simulink model "pid_controller_pitch"  (R2023a)
settings: Solver=FixedStepAuto  StartTime=0.0  StopTime=inf  FixedStep=Ts_slk  RelTol=1e-3  EnableMultiTasking=on
undefined symbols (not defined in the file): A_cond, B_cond, C, D, dev, IMU_w_b_bias, K, Main, meas_pole, P0_phth, P0_ps, prefilter_pole, pwm_output0, Q_phth, q_ps, R_phth, r_ps, Rz, Ts_EKF_integr, Ts_EKF_meas, Ts_slk, x0_phth, x0_ps
libraries: px4Sensorslib x4, slpidlib x2, cstblocks x1, px4lib x1, px4uORBlib x1, sharedtransform x1
(part 1 of 2)
settings Model: ExtModeTrigDuration=10  Creator=ArriGE66  LastModifiedBy=User
settings SolverCC: PositivePriorityOrder=on
settings OptimizationCC: EnhancedBackFolding=on  PassReuseOutputArgsAs=Individual arguments  ZeroExternalMemoryAtStartup=off  ZeroInternalMemoryAtStartup=off  MaxStackSize=64  OptimizeBlockOrder=speed  DifferentSizesBufferReuse=on  OptimizationCustomize=off  EfficientTunableParamExpr=on
settings DebuggingCC: ParameterTunabilityLossMsg=error
settings HardwareCC: ProdBitPerPointer=32  ProdBitPerSizeT=32  ProdBitPerPtrDiffT=32  ProdLargestAtomicInteger=Long  ProdLargestAtomicFloat=Double  ProdWordSize=32  ProdLongLongMode=on  ProdHWDeviceType=ARM Compatible->ARM Cortex
settings SFSimCC: MATLABDynamicMemAlloc=off  SimTargetLang=C++
settings RTWCC: Description=Embedded Coder  SystemTargetFile=ert.tlc  HardwareBoard=PX4 Cube Orange  TLCOptions="-aInlineSetEventsForThisBaseRateFcn=TLC_FALSE -aSuppressMultiTaskScheduler=TLC_FALSE  -aRateBasedStepFcn=0"  TemplateMakefile=ert_default_tmf  Toolchain=GNU Tools for PX4 Autopilots  TargetLang=C++
settings CodeAppCC: ForceParamTrailComments=on  IgnoreCustomStorageClasses=off  OperatorAnnotations=on  SimulinkDataObjDesc=on  SFDataObjDesc=on  InsertBlockDesc=on
settings ERTTargetCC: ExtModeTransport=3  ExtModeStaticAlloc=on  ExtModeStaticAllocSize=1024  ExtModeMexFile=ext_xcp  ExtModeIntrfLevel=Level2 - Open

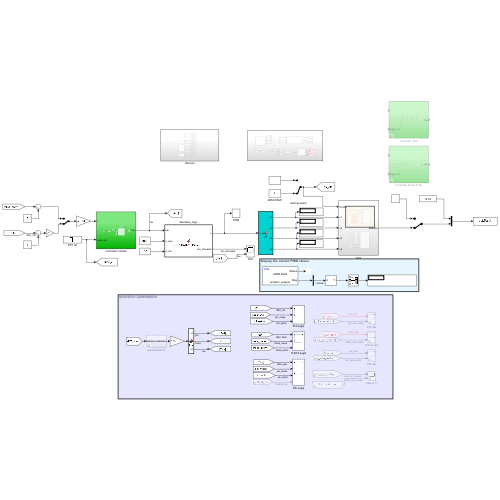
[thumbnail: Simulink's stored preview of the top-level diagram]
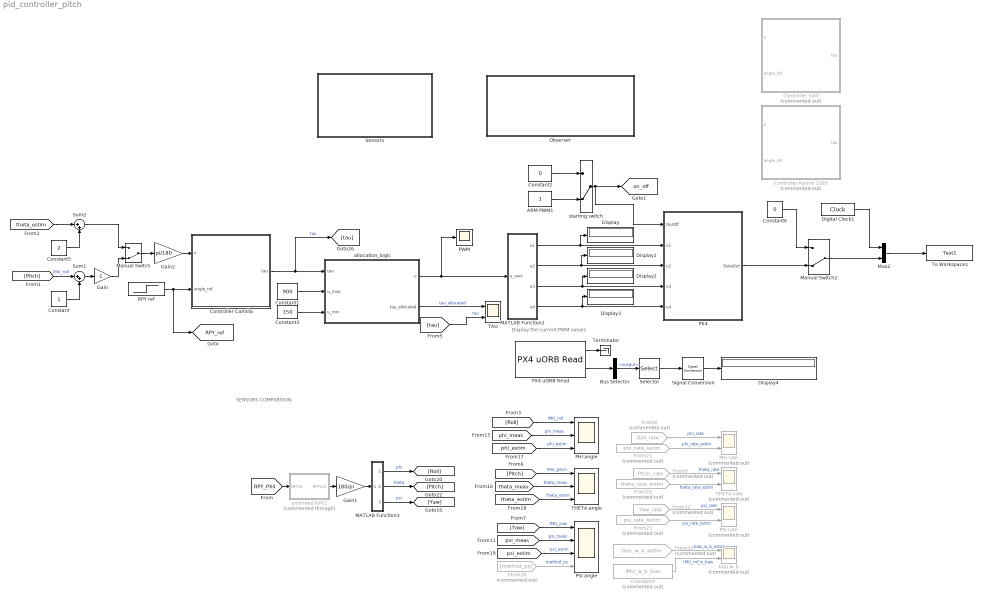
== system pid_controller_pitch ==
  note: Display the current PWM values
  note: SENSORS COMPARISON
  ARM PWM1 : Constant  OutDataTypeStr=boolean  SampleTime=Ts_slk
  Bus Selector : BusSelector  OutputSignals=output
  Constant : Constant  SampleTime=0.01
  Constant1 : Constant  Value=900  SampleTime=0.01
  Constant2 : Constant  Value=0  OutDataTypeStr=boolean
  Constant3 : Constant  Value=150  SampleTime=0.01
  Constant4 : Constant  Commented=on  Value=IMU_w_b_bias
  Constant5 : Constant  Value=2  SampleTime=0.01
  Constant6 : Constant  Value=0  OutDataTypeStr=boolean
  Controller 1dof : Subsystem  Commented=on
  Controller Camilla : Subsystem
  Controller Karimi 2105 : Subsystem  Commented=on
  Digital Clock1 : DigitalClock  SampleTime=0.01
  Display{,1..4} (5 alike) : Display
  From12 : From  Commented=on  GotoTag=Yaw_rate  TagVisibility=global
  From20 : From  Commented=on  GotoTag=method_ps
  From21 : From  Commented=on  GotoTag=phi_rate_estim
  From22 : From  Commented=on  GotoTag=theta_rate_estim
  From23 : From  Commented=on  GotoTag=psi_rate_estim
  From24 : From  Commented=on  GotoTag=bias_w_b_estim
  From8 : From  Commented=on  GotoTag=Roll_rate  TagVisibility=global
  From9 : From  Commented=on  GotoTag=Pitch_rate  TagVisibility=global
  Gain : Gain  Gain=-1
  Gain1 : Gain  Gain=180/pi
  Gain2 : Gain  Gain=pi/180
  MATLAB Function2 : MATLAB Function  TreatAsAtomicUnit=on
  MATLAB Function3 : MATLAB Function  TreatAsAtomicUnit=on
  Manual Switch : ManualSwitch  CurrentSetting=0
  Manual Switch2 : ManualSwitch  CurrentSetting=0
  Mux2 : Mux  Inputs=2
  Observer : Subsystem
  PHI angle : Scope  NumInputPorts=3
  PHI rate : Scope  Commented=on  NumInputPorts=2
  PSI angle : Scope  NumInputPorts=4
  PSI rate : Scope  Commented=on  NumInputPorts=2
  PWM : Scope
  PX4 : Subsystem
  PX4 uORB Read : px4uORBlib/PX4 uORB Read  uORBTopic=actuator_outputs  selectInstance=actuator_outputs  SampleTime=0.01  BlockingMode=off  BlockTimeout=1e-3
  RPY ref : Step  Time=0  After=pi/180*(-4)  SampleTime=Ts_slk
  Selector : Selector  InputPortWidth=16  IndexOptions=Index vector (dialog)  Indices=[1 2 3 4]  OutputSizes=1
  Sensors : Subsystem
  Signal Conversion : SignalConversion  OverrideOpt=off
  Sum1 : Sum  Inputs=|++
  Sum2 : Sum  Inputs=|++
  TAU : Scope  NumInputPorts=2
  THETA angle : Scope  NumInputPorts=3
  THETA rate : Scope  Commented=on  NumInputPorts=2
  Terminator : Terminator
  To Workspace1 : ToWorkspace  VariableName=Test1  SampleTime=-1
      settings: Save2DSignal=2-D array (concatenate along first dimension)
  allocation_logic : MATLAB Function  TreatAsAtomicUnit=on
  bias w_b : Scope  Commented=on  NumInputPorts=2
  starting switch : ManualSwitch  CurrentSetting=0
  unlimited RPY2 : Subsystem  Commented=through
  tag scope: RPY_ref=global, on_off=global
  wires:
  Manual Switch/1 -> Gain2/1
  MATLAB Function2/4(u4) -> PX4/5(u4), Display3/1
  Constant5/1 -> Sum2/2
  Constant4/1 -> bias w_b/2  "IMU_mf_b_bias"
  From8/1 -> PHI rate/1  "phi_rate"
  [RPY_PX4] -> unlimited RPY2/1(RPYin)
  Constant1/1 -> allocation_logic/2(u_max)
  PX4/1(DataOut) -> Manual Switch2/2
  Constant/1 -> Sum1/2
  PX4 uORB Read/2 -> Bus Selector/1
  From22/1 -> THETA rate/2  "theta_rate_estim"
  RPY ref/1 -> [RPY_ref], Controller Camilla/2(angle_ref)
  [theta_estim] -> Sum2/1
  allocation_logic/1(u) -> PWM/1, MATLAB Function2/1(u_vect)
  From21/1 -> PHI rate/2  "phi_rate_estim"
  [phi_meas] -> PHI angle/2  "phi_meas"
  [theta_meas] -> THETA angle/2  "theta_meas"
  unlimited RPY2/1(RPYout) -> Gain1/1
  Constant6/1 -> Manual Switch2/1
  [Roll] -> PHI angle/1  "IMU_roll"
  From23/1 -> PSI rate/2  "psi_rate_estim"
  Selector/1 -> Signal Conversion/1
  [psi_estim] -> PSI angle/3  "psi_estim"
  [theta_estim] -> THETA angle/3  "theta_estim"
  MATLAB Function3/2(y2) -> [Pitch]  "theta"
  Manual Switch2/1 -> Mux2/2
  Sum2/1 -> Manual Switch/1
  [psi_meas] -> PSI angle/2  "psi_meas"
  From20/1 -> PSI angle/4  "method_ps"
  [phi_estim] -> PHI angle/3  "phi_estim"
  Signal Conversion/1 -> Display4/1
  Bus Selector/1 -> Selector/1  "<output>"
  starting switch/1 -> PX4/1(On/Off), [on_off]
  [Pitch] -> THETA angle/1  "IMU_pitch"
  [Yaw] -> PSI angle/1  "IMU_yaw"
  MATLAB Function2/3(u3) -> PX4/4(u3), Display2/1
  From9/1 -> THETA rate/1  "theta_rate"
  Controller Camilla/1(tau) -> [tau], allocation_logic/1(tau)  "tau"
  ARM PWM1/1 -> starting switch/2
  Mux2/1 -> To Workspace1/1
  MATLAB Function3/3(y3) -> [Yaw]  "psi"
  Gain1/1 -> MATLAB Function3/1(u)
  MATLAB Function2/1(u1) -> Display/1, PX4/2(u1)
  [Pitch] -> Sum1/1  "IMU_roll"
  From12/1 -> PSI rate/1  "psi_rate"
  Digital Clock1/1 -> Mux2/1
  allocation_logic/2(tau_allocated) -> TAU/1  "tau_allocated"
  MATLAB Function3/1(y1) -> [Roll]  "phi"
  Sum1/1 -> Gain/1
  Constant3/1 -> allocation_logic/3(u_min)
  [tau] -> TAU/2  "tau"
  MATLAB Function2/2(u2) -> Display1/1, PX4/3(u2)
  From24/1 -> bias w_b/1  "bias_w_b_estim"
  Gain2/1 -> Controller Camilla/1(x)
  Constant2/1 -> starting switch/1
  PX4 uORB Read/1 -> Terminator/1
  Gain/1 -> Manual Switch/2

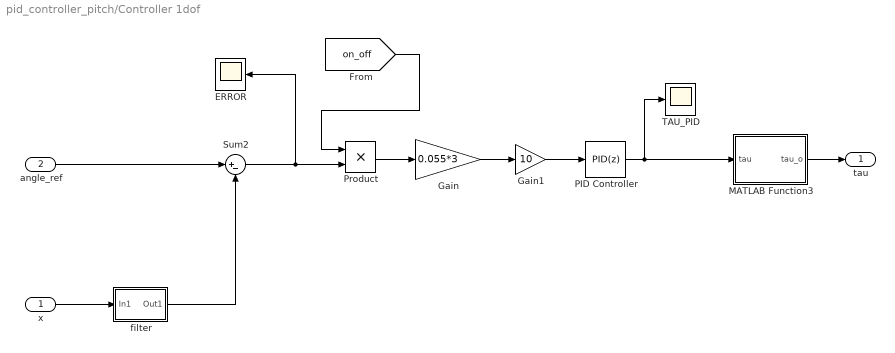
== system pid_controller_pitch/Controller 1dof ==
  x : Inport
  angle_ref : Inport  Port=2
  ERROR : Scope
  Gain : Gain  Gain=0.055*3
  Gain1 : Gain  Gain=10
  MATLAB Function3 : MATLAB Function  TreatAsAtomicUnit=on
  PID Controller : slpidlib/PID Controller  Controller=PID  Form=Parallel  TimeDomain=Discrete-time  UseExternalTs=off  SampleTime=Ts_slk  IntegratorMethod=Forward Euler  FilterMethod=Forward Euler  ControllerParametersSource=internal  P=0.01  I=0  UseKiTs=off  D=1  N=100  UseFilter=on  TunerSelectOption=Transfer Function Based (PID Tuner App)  InitialConditionSource=internal  InitialConditionForIntegrator=0  InitialConditionForFilter=0  DifferentiatorICPrevScaledInput=0  ExternalReset=none  TrackingMode=off  Kt=1  LimitOutput=on  SatLimitsSource=internal  UpperSaturationLimit=1.29  LowerSaturationLimit=-1.29  LinearizeAsGain=on  AntiWindupMode=clamping  Kb=1  LimitIntegrator=off  UpperIntegratorSaturationLimit=inf  LowerIntegratorSaturationLimit=-inf  POutMin=[]  POutMax=[]  IOutMin=[]  IOutMax=[]  DOutMin=[]  DOutMax=[]  NOutMin=[]  NOutMax=[]  SumOutMin=[]  SumOutMax=[]  SaturationOutMin=[]  SaturationOutMax=[]  PParamMin=[]  PParamMax=[]  IParamMin=[]  IParamMax=[]  DParamMin=[]  DParamMax=[]  NParamMin=[]  NParamMax=[]  KbParamMin=[]  KbParamMax=[]  KtParamMin=[]  KtParamMax=[]  KbOutMin=[]  KbOutMax=[]  KtOutMin=[]  KtOutMax=[]  IntegratorOutMin=[]  IntegratorOutMax=[]  FilterOutMin=[]  FilterOutMax=[]  SumI1OutMin=[]  SumI1OutMax=[]  SumI2OutMin=[]  SumI2OutMax=[]  SumI3OutMin=[]  SumI3OutMax=[]  SumI4OutMin=[]  SumI4OutMax=[]  SumDOutMin=[]  SumDOutMax=[]  DifferentiatorOutMin=[]  DifferentiatorOutMax=[]  FilterDiffOutCoefMin=[]  FilterDiffOutCoefMax=[]  ReciprocalOutMin=[]  ReciprocalOutMax=[]  SumDenOutMin=[]  SumDenOutMax=[]  SumNumOutMin=[]  SumNumOutMax=[]  DivideOutMin=[]  DivideOutMax=[]  UdiffTsProdOutMin=[]  UdiffTsProdOutMax=[]  NTsProdOutMin=[]  NTsProdOutMax=[]  UintegralTsProdOutMin=[]  UintegralTsProdOutMax=[]  UngainTsProdOutMin=[]  UngainTsProdOutMax=[]  ClampingZeroOutDataTypeStr=Inherit: Inherit via back propagation  ClampingZeroOutMin=[]  ClampingZeroOutMax=[]  FilterDenConstantOutDataTypeStr=Inherit: Inherit via back propagation  FilterDenConstantOutMin=[]  FilterDenConstantOutMax=[]  PCopyOutDataTypeStr=Inherit: Inherit via back propagation  PCopyOutMin=[]  PCopyOutMax=[]  NCopyOutDataTypeStr=Inherit: Inherit via back propagation  NCopyOutMin=[]  NCopyOutMax=[]  IntegratorContinuousStateAttributes=''  IntegratorStateMustResolveToSignalObject=off  IntegratorRTWStateStorageClass=Auto  FilterContinuousStateAttributes=''  FilterStateMustResolveToSignalObject=off  FilterRTWStateStorageClass=Auto  ParallelPVariant=InternalParameters  IdealPVariant=Disabled  IVariant=InternalParameters  DVariant=InternalParameters  IntegratorVariant=Discrete  SatVariant=Enabled  AWVariant=DiscClampingParallel  PCopyVariant=Disabled  TRVariant=Disabled  FdbkBlocksVariant=Forward  IdealPFdbkVariant=Disabled  SatFdbkVariant=Disabled  DerivativeFilterVariant=ForwardEulerFilter  NVariant=InternalParameters  NCopyVariant=Disabled  FilterICVariant=InternalICsFilter  IntegratorICVariant=InternalICs  ExternalResetVariant=Disabled  TRSumVariant=Passthrough  SumFdbkVariant=Disabled  SumVariant=Sum_PID  TsampFilterVariant=InternalTs  TsampNgainVariant=Passthrough  TsampIntegralVariant=Disabled_SignalSpec  ExternalSaturationOutDataTypeStr=Inherit: Same as second input
  Product : Product
  Sum2 : Sum  Inputs=|+-
  TAU_PID : Scope
  filter : Subsystem  mask{p=meas_pole}
      mask prompts: p "pole (p)"
  tau : Outport
  wires:
  angle_ref/1 -> Sum2/1
  MATLAB Function3/1(tau_o) -> tau/1
  Sum2/1 -> ERROR/1, Product/2
  x/1 -> filter/1(In1)
  Product/1 -> Gain/1
  [on_off] -> Product/1
  PID Controller/1 -> MATLAB Function3/1(tau), TAU_PID/1
  filter/1(Out1) -> Sum2/2
  Gain/1 -> Gain1/1
  Gain1/1 -> PID Controller/1

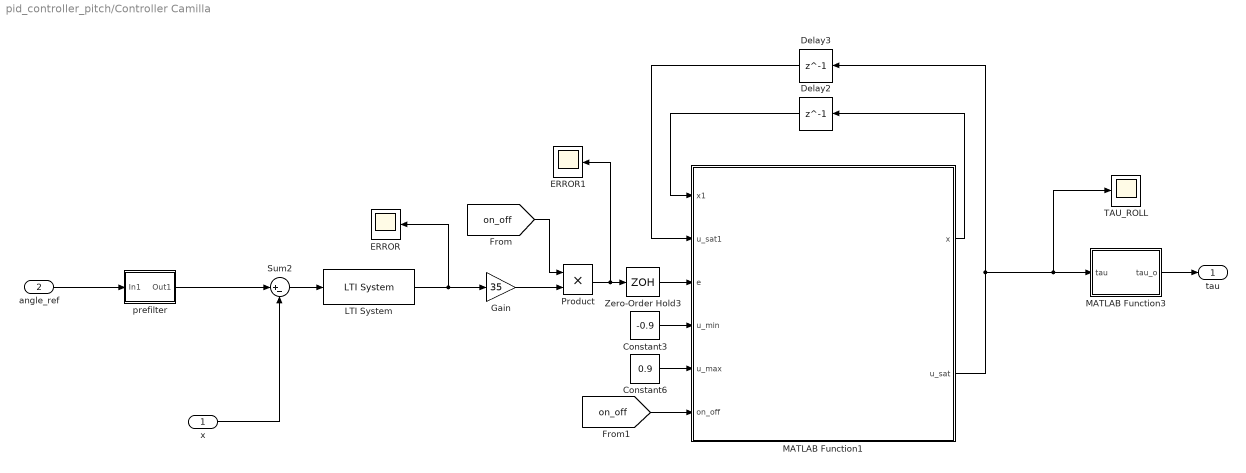
== system pid_controller_pitch/Controller Camilla ==
  x : Inport
  angle_ref : Inport  Port=2
  " prefilter" : Subsystem  mask{p=prefilter_pole}
      mask prompts: p "pole (p)"
  Constant3 : Constant  Value=-0.9  SampleTime=Ts_slk
  Constant6 : Constant  Value=0.9  SampleTime=Ts_slk
  Delay2 : Delay  DelayLength=1  InitialCondition=zeros(2,1)  SampleTime=Ts_slk
  Delay3 : Delay  DelayLength=1  InitialCondition=0  SampleTime=Ts_slk
  ERROR : Scope
  ERROR1 : Scope
  Gain : Gain  Gain=35
  LTI System : cstblocks/LTI System  sys=filter_d  IC=[]
  MATLAB Function1 : MATLAB Function  TreatAsAtomicUnit=on
  MATLAB Function3 : MATLAB Function  TreatAsAtomicUnit=on
  Product : Product
  Sum2 : Sum  Inputs=|+-
  TAU_ROLL : Scope
  Zero-Order Hold3 : ZeroOrderHold  SampleTime=Ts_slk
  tau : Outport
  wires:
  angle_ref/1 -> " prefilter"/1(In1)
  MATLAB Function3/1(tau_o) -> tau/1
  Sum2/1 -> LTI System/1
  MATLAB Function1/2(u_sat) -> TAU_ROLL/1, MATLAB Function3/1(tau), Delay3/1
  Product/1 -> ERROR1/1, Zero-Order Hold3/1
  [on_off] -> Product/1
  x/1 -> Sum2/2
  Constant6/1 -> MATLAB Function1/5(u_max)
  Zero-Order Hold3/1 -> MATLAB Function1/3(e)
  MATLAB Function1/1(x) -> Delay2/1
  Delay3/1 -> MATLAB Function1/2(u_sat1)
  Constant3/1 -> MATLAB Function1/4(u_min)
  Delay2/1 -> MATLAB Function1/1(x1)
  Gain/1 -> Product/2
  [on_off] -> MATLAB Function1/6(on_off)
  LTI System/1 -> ERROR/1, Gain/1
  " prefilter"/1(Out1) -> Sum2/1

== system pid_controller_pitch/Controller Karimi 2105 ==
  x : Inport
  angle_ref : Inport  Port=2
  Gain : Gain  Gain=K
  MATLAB Function3 : MATLAB Function  TreatAsAtomicUnit=on
  PID Controller2 : slpidlib/PID Controller  Controller=PID  Form=Parallel  TimeDomain=Discrete-time  UseExternalTs=off  SampleTime=Ts_slk  IntegratorMethod=Forward Euler  FilterMethod=Forward Euler  ControllerParametersSource=internal  P=0.180109037198918  I=0.150719618455462  UseKiTs=off  D=0.0291322547663788  N=114.28279760416  UseFilter=on  TunerSelectOption=Transfer Function Based (PID Tuner App)  InitialConditionSource=internal  InitialConditionForIntegrator=0  InitialConditionForFilter=0  DifferentiatorICPrevScaledInput=0  ExternalReset=none  TrackingMode=off  Kt=1  LimitOutput=on  SatLimitsSource=internal  UpperSaturationLimit=1.2  LowerSaturationLimit=-1.2  LinearizeAsGain=on  AntiWindupMode=clamping  Kb=1  LimitIntegrator=off  UpperIntegratorSaturationLimit=inf  LowerIntegratorSaturationLimit=-inf  POutMin=[]  POutMax=[]  IOutMin=[]  IOutMax=[]  DOutMin=[]  DOutMax=[]  NOutMin=[]  NOutMax=[]  SumOutMin=[]  SumOutMax=[]  SaturationOutMin=[]  SaturationOutMax=[]  PParamMin=[]  PParamMax=[]  IParamMin=[]  IParamMax=[]  DParamMin=[]  DParamMax=[]  NParamMin=[]  NParamMax=[]  KbParamMin=[]  KbParamMax=[]  KtParamMin=[]  KtParamMax=[]  KbOutMin=[]  KbOutMax=[]  KtOutMin=[]  KtOutMax=[]  IntegratorOutMin=[]  IntegratorOutMax=[]  FilterOutMin=[]  FilterOutMax=[]  SumI1OutMin=[]  SumI1OutMax=[]  SumI2OutMin=[]  SumI2OutMax=[]  SumI3OutMin=[]  SumI3OutMax=[]  SumI4OutMin=[]  SumI4OutMax=[]  SumDOutMin=[]  SumDOutMax=[]  DifferentiatorOutMin=[]  DifferentiatorOutMax=[]  FilterDiffOutCoefMin=[]  FilterDiffOutCoefMax=[]  ReciprocalOutMin=[]  ReciprocalOutMax=[]  SumDenOutMin=[]  SumDenOutMax=[]  SumNumOutMin=[]  SumNumOutMax=[]  DivideOutMin=[]  DivideOutMax=[]  UdiffTsProdOutMin=[]  UdiffTsProdOutMax=[]  NTsProdOutMin=[]  NTsProdOutMax=[]  UintegralTsProdOutMin=[]  UintegralTsProdOutMax=[]  UngainTsProdOutMin=[]  UngainTsProdOutMax=[]  ClampingZeroOutDataTypeStr=Inherit: Inherit via back propagation  ClampingZeroOutMin=[]  ClampingZeroOutMax=[]  FilterDenConstantOutDataTypeStr=Inherit: Inherit via back propagation  FilterDenConstantOutMin=[]  FilterDenConstantOutMax=[]  PCopyOutDataTypeStr=Inherit: Inherit via back propagation  PCopyOutMin=[]  PCopyOutMax=[]  NCopyOutDataTypeStr=Inherit: Inherit via back propagation  NCopyOutMin=[]  NCopyOutMax=[]  IntegratorContinuousStateAttributes=''  IntegratorStateMustResolveToSignalObject=off  IntegratorRTWStateStorageClass=Auto  FilterContinuousStateAttributes=''  FilterStateMustResolveToSignalObject=off  FilterRTWStateStorageClass=Auto  ParallelPVariant=InternalParameters  IdealPVariant=Disabled  IVariant=InternalParameters  DVariant=InternalParameters  IntegratorVariant=Discrete  SatVariant=Enabled  AWVariant=DiscClampingParallel  PCopyVariant=Disabled  TRVariant=Disabled  FdbkBlocksVariant=Forward  IdealPFdbkVariant=Disabled  SatFdbkVariant=Disabled  DerivativeFilterVariant=ForwardEulerFilter  NVariant=InternalParameters  NCopyVariant=Disabled  FilterICVariant=InternalICsFilter  IntegratorICVariant=InternalICs  ExternalResetVariant=Disabled  TRSumVariant=Passthrough  SumFdbkVariant=Disabled  SumVariant=Sum_PID  TsampFilterVariant=InternalTs  TsampNgainVariant=Passthrough  TsampIntegralVariant=Disabled_SignalSpec  ExternalSaturationOutDataTypeStr=Inherit: Same as second input
  PID with saturation4 : Subsystem
  Sum : Sum  Inputs=|+-
  Sum1 : Sum  Inputs=|++
  filter : Subsystem  mask{p=meas_pole}
      mask prompts: p "pole (p)"
  tau : Outport
  wires:
  Sum/1 -> PID Controller2/1
  PID Controller2/1 -> MATLAB Function3/1(tau)
  filter/1(Out1) -> Sum/2
  angle_ref/1 -> Sum/1
  x/1 -> Gain/1, filter/1(In1)
  MATLAB Function3/1(tau_o) -> Sum1/1
  Sum1/1 -> tau/1
  Gain/1 -> Sum1/2

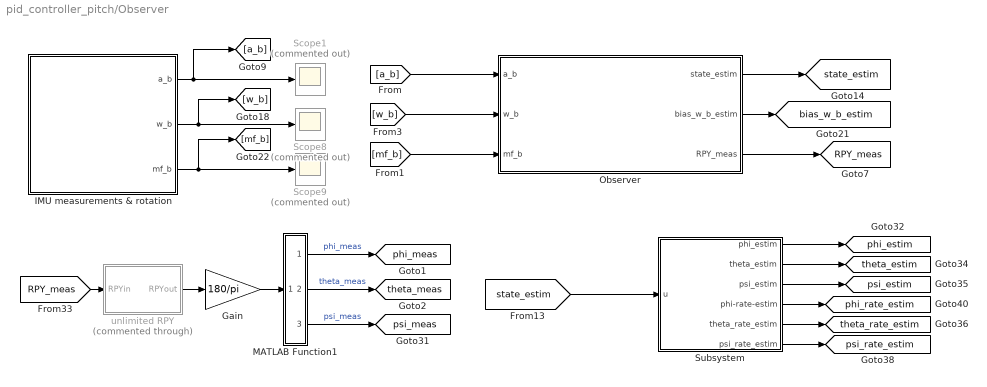
== system pid_controller_pitch/Observer ==
  Gain : Gain  Gain=180/pi
  IMU measurements & rotation : Subsystem
  MATLAB Function1 : MATLAB Function  TreatAsAtomicUnit=on
  Observer : Subsystem
  Scope1 : Scope  Commented=on
  Scope8 : Scope  Commented=on
  Scope9 : Scope  Commented=on
  Subsystem : Subsystem
  unlimited RPY : Subsystem  Commented=through
  tag scope: RPY_meas=global, bias_w_b_estim=global, phi_estim=global, phi_meas=global, phi_rate_estim=global, psi_estim=global, psi_meas=global, psi_rate_estim=global, state_estim=global, theta_estim=global, theta_meas=global, theta_rate_estim=global
  wires:
  MATLAB Function1/1(y1) -> [phi_meas]  "phi_meas"
  [w_b] -> Observer/2(w_b)
  Subsystem/6(psi_rate_estim) -> [psi_rate_estim]
  IMU measurements & rotation/1(a_b) -> [a_b], Scope1/1
  Subsystem/5(theta_rate_estim) -> [theta_rate_estim]
  Observer/2(bias_w_b_estim) -> [bias_w_b_estim]
  Observer/1(state_estim) -> [state_estim]
  [state_estim] -> Subsystem/1(u)
  MATLAB Function1/2(y2) -> [theta_meas]  "theta_meas"
  Observer/3(RPY_meas) -> [RPY_meas]
  [a_b] -> Observer/1(a_b)
  Subsystem/4(phi-rate-estim) -> [phi_rate_estim]
  [RPY_meas] -> unlimited RPY/1(RPYin)
  [mf_b] -> Observer/3(mf_b)
  Subsystem/3(psi_estim) -> [psi_estim]
  unlimited RPY/1(RPYout) -> Gain/1
  Subsystem/2(theta_estim) -> [theta_estim]
  Subsystem/1(phi_estim) -> [phi_estim]
  Gain/1 -> MATLAB Function1/1(u)
  MATLAB Function1/3(y3) -> [psi_meas]  "psi_meas"
  IMU measurements & rotation/3(mf_b) -> [mf_b], Scope9/1
  IMU measurements & rotation/2(w_b) -> [w_b], Scope8/1

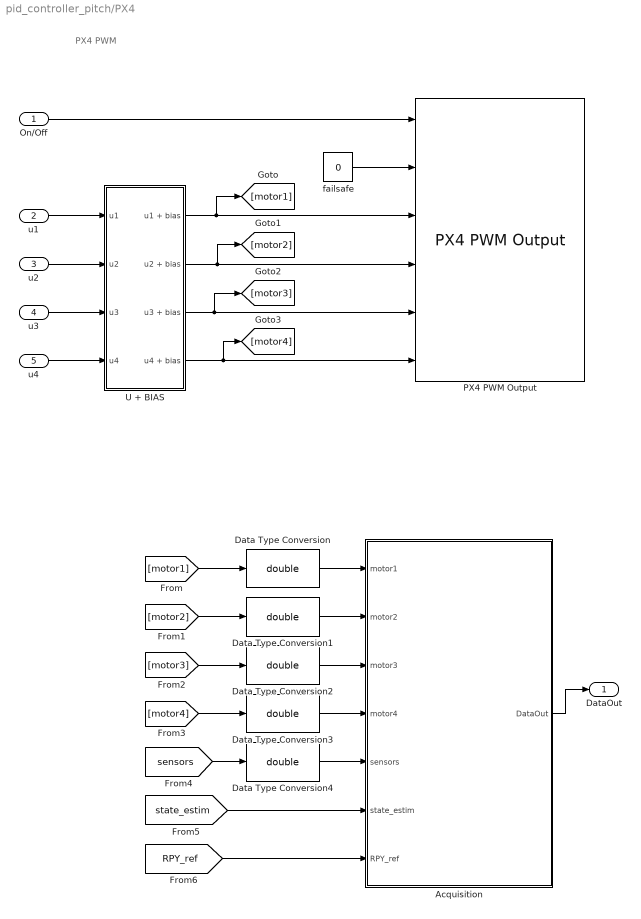
== system pid_controller_pitch/PX4 ==
  note: PX4 PWM
  On/Off : Inport
  u1 : Inport  Port=2
  u2 : Inport  Port=3
  u3 : Inport  Port=4
  u4 : Inport  Port=5
  Acquisition : Subsystem
  Data Type Conversion{,1..4} (5 alike) : DataTypeConversion  OutDataTypeStr=double  RndMeth=Nearest  SaturateOnIntegerOverflow=off
  PX4 PWM Output : px4lib/PX4 PWM Output  pwmDevice=Main (/dev/pwm_output0)  pwmChannel1_=on  pwmChannel2_=on  pwmChannel3_=on  pwmChannel4_=on  pwmChannel5_=off  pwmChannel6_=off  pwmChannel7_=off  pwmChannel8_=off  forceTerminateFailsafe=off  outputErrorStatus=off
  U + BIAS : Subsystem
  failsafe : Constant  Value=0  OutDataTypeStr=boolean  SampleTime=0.01
  DataOut : Outport
  wires:
  On/Off/1 -> PX4 PWM Output/1
  u1/1 -> U + BIAS/1(u1)
  u2/1 -> U + BIAS/2(u2)
  u4/1 -> U + BIAS/4(u4)
  u3/1 -> U + BIAS/3(u3)
  failsafe/1 -> PX4 PWM Output/2
  U + BIAS/1(u1 + bias) -> [motor1], PX4 PWM Output/3
  U + BIAS/2(u2 + bias) -> PX4 PWM Output/4, [motor2]
  U + BIAS/3(u3 + bias) -> PX4 PWM Output/5, [motor3]
  U + BIAS/4(u4 + bias) -> [motor4], PX4 PWM Output/6
  [sensors] -> Data Type Conversion4/1
  [motor1] -> Data Type Conversion/1
  [motor2] -> Data Type Conversion1/1
  [motor3] -> Data Type Conversion2/1
  [motor4] -> Data Type Conversion3/1
  [state_estim] -> Acquisition/6(state_estim)
  Acquisition/1(DataOut) -> DataOut/1
  Data Type Conversion/1 -> Acquisition/1(motor1)
  Data Type Conversion1/1 -> Acquisition/2(motor2)
  Data Type Conversion2/1 -> Acquisition/3(motor3)
  Data Type Conversion3/1 -> Acquisition/4(motor4)
  Data Type Conversion4/1 -> Acquisition/5(sensors)
  [RPY_ref] -> Acquisition/7(RPY_ref)

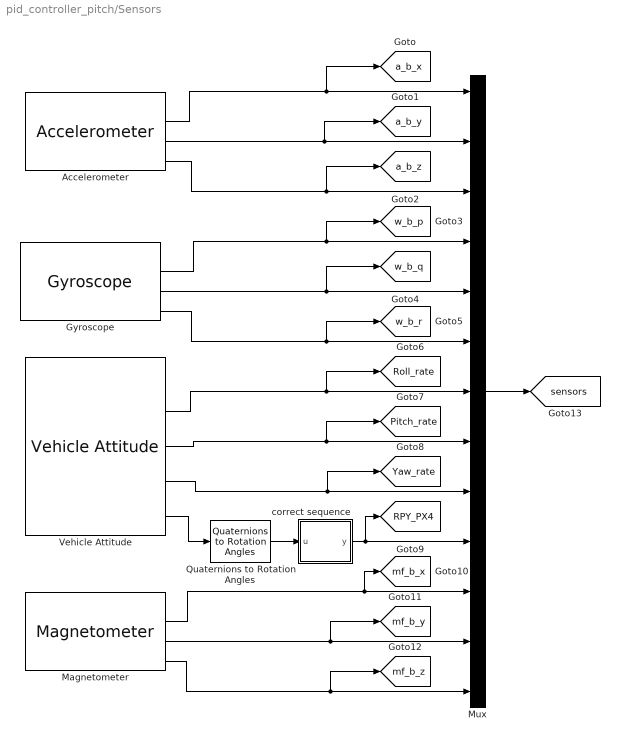
== system pid_controller_pitch/Sensors ==
  Accelerometer : px4Sensorslib/Accelerometer  uorbTimeStamp=off  BlockingMode=off  BlockTimeout=1e-3  sampleTime=1/100
  Gyroscope : px4Sensorslib/Gyroscope  uorbTimeStamp=off  BlockingMode=off  BlockTimeout=1e-3  sampleTime=1/100
  Magnetometer : px4Sensorslib/Magnetometer  uorbTimeStamp=off  BlockingMode=off  BlockTimeout=1e-3  sampleTime=1/100
  Mux : Mux  Inputs=13
  Quaternions to Rotation Angles : sharedtransform/Quaternions to Rotation Angles  rotationOrder=ZYX  aMode=aMode
  Vehicle Attitude : px4Sensorslib/Vehicle Attitude  rollRate=on  pitchRate=on  yawRate=on  quaternion=on  uorbTimeStamp=off  BlockingMode=off  BlockTimeout=0.001  sampleTime=1/100
  correct sequence : MATLAB Function  TreatAsAtomicUnit=on
  tag scope: Pitch_rate=global, RPY_PX4=global, Roll_rate=global, Yaw_rate=global, a_b_x=global, a_b_y=global, a_b_z=global, mf_b_x=global, mf_b_y=global, mf_b_z=global, sensors=global, w_b_p=global, w_b_q=global, w_b_r=global
  wires:
  Vehicle Attitude/3 -> Mux/8, [Pitch_rate]
  Magnetometer/4 -> [mf_b_z], Mux/13
  Quaternions to Rotation Angles/1 -> correct sequence/1(u)
  Gyroscope/2 -> Mux/4, [w_b_p]
  Magnetometer/3 -> [mf_b_y], Mux/12
  Accelerometer/2 -> Mux/1, [a_b_x]
  Vehicle Attitude/4 -> Mux/9, [Yaw_rate]
  Accelerometer/3 -> [a_b_y], Mux/2
  Vehicle Attitude/2 -> Mux/7, [Roll_rate]
  correct sequence/1(y) -> [RPY_PX4], Mux/10
  Gyroscope/4 -> Mux/6, [w_b_r]
  Magnetometer/2 -> Mux/11, [mf_b_x]
  Accelerometer/4 -> Mux/3, [a_b_z]
  Vehicle Attitude/5 -> Quaternions to Rotation Angles/1
  Gyroscope/3 -> Mux/5, [w_b_q]
  Mux/1 -> [sensors]

== system pid_controller_pitch/unlimited RPY2 ==
  RPYin : Inport
  Memory : Memory
  Memory1 : Memory
  unlimited RPY : MATLAB Function  TreatAsAtomicUnit=on
  RPYout : Outport
  wires:
  RPYin/1 -> unlimited RPY/1("RPY ")
  unlimited RPY/1(RPY) -> Memory/1, RPYout/1
  Memory/1 -> unlimited RPY/2(RPY1)
  unlimited RPY/2(init) -> Memory1/1
  Memory1/1 -> unlimited RPY/3("init ")

== system pid_controller_pitch/Controller 1dof/filter ==
  In1 : Inport
  Discrete Transfer Fcn2 : DiscreteTransferFcn  Numerator=[Ts_slk*p]  Denominator=[1 (Ts_slk*p-1)]
  Transfer Fcn1 : TransferFcn  Commented=on  Denominator=[1/p 1]
  Out1 : Outport
  wires:
  In1/1 -> Discrete Transfer Fcn2/1
  Discrete Transfer Fcn2/1 -> Out1/1

== system pid_controller_pitch/Controller Camilla/ prefilter ==
  In1 : Inport
  Discrete Transfer Fcn1 : DiscreteTransferFcn  Numerator=[Ts_slk*p]  Denominator=[1 (Ts_slk*p-1)]
  Transfer Fcn1 : TransferFcn  Commented=on  Denominator=[1/p 1]
  Out1 : Outport
  wires:
  In1/1 -> Discrete Transfer Fcn1/1
  Discrete Transfer Fcn1/1 -> Out1/1

== system pid_controller_pitch/Controller Karimi 2105/PID with saturation4 ==
  In1 : Inport
  Delay : Delay  DelayLength=1
  Delay1 : Delay  DelayLength=1
  Gain2 : Gain
  Ki : Gain  Gain=-10*Ts_slk
  Kp : Gain  Gain=0.2
  Saturation : Saturate  UpperLimit=1.0267  LowerLimit=-1.0267
  Sum : Sum  Inputs=+++
  Sum2 : Sum  Inputs=++|
  Sum3 : Sum  Inputs=-+
  tau : Outport
  wires:
  In1/1 -> Ki/1, Kp/1
  Sum2/1 -> Sum3/1, Saturation/1
  Sum3/1 -> Delay1/1
  Saturation/1 -> tau/1, Sum3/2
  Kp/1 -> Sum2/1
  Sum/1 -> Sum2/2, Delay/1
  Gain2/1 -> Sum/3
  Ki/1 -> Sum/2
  Delay/1 -> Sum/1
  Delay1/1 -> Gain2/1

== system pid_controller_pitch/Controller Karimi 2105/filter ==
  In1 : Inport
  Discrete Transfer Fcn2 : DiscreteTransferFcn  Numerator=[Ts_slk*p]  Denominator=[1 (Ts_slk*p-1)]
  Transfer Fcn1 : TransferFcn  Commented=on  Denominator=[1/p 1]
  Out1 : Outport
  wires:
  In1/1 -> Discrete Transfer Fcn2/1
  Discrete Transfer Fcn2/1 -> Out1/1

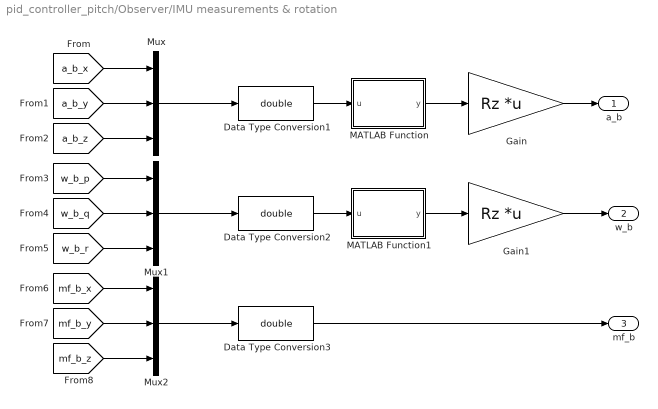
== system pid_controller_pitch/Observer/IMU measurements & rotation ==
  Data Type Conversion1 : DataTypeConversion  OutDataTypeStr=double  SaturateOnIntegerOverflow=off  RndMeth=Floor
  Data Type Conversion2 : DataTypeConversion  OutDataTypeStr=double  SaturateOnIntegerOverflow=off  RndMeth=Floor
  Data Type Conversion3 : DataTypeConversion  OutDataTypeStr=double  SaturateOnIntegerOverflow=off  RndMeth=Floor
  Gain : Gain  Gain=Rz  Multiplication=Matrix(K*u) (u vector)
  Gain1 : Gain  Gain=Rz  Multiplication=Matrix(K*u) (u vector)
  MATLAB Function : MATLAB Function  TreatAsAtomicUnit=on
  MATLAB Function1 : MATLAB Function  TreatAsAtomicUnit=on
  Mux : Mux  Inputs=3
  Mux1 : Mux  Inputs=3
  Mux2 : Mux  Inputs=3
  a_b : Outport
  w_b : Outport  Port=2
  mf_b : Outport  Port=3
  wires:
  [w_b_p] -> Mux1/1
  Data Type Conversion3/1 -> mf_b/1
  Data Type Conversion2/1 -> MATLAB Function1/1(u)
  [mf_b_y] -> Mux2/2
  Mux1/1 -> Data Type Conversion2/1
  Mux/1 -> Data Type Conversion1/1
  [a_b_y] -> Mux/2
  Mux2/1 -> Data Type Conversion3/1
  [w_b_q] -> Mux1/2
  [mf_b_z] -> Mux2/3
  [a_b_z] -> Mux/3
  [a_b_x] -> Mux/1
  [mf_b_x] -> Mux2/1
  [w_b_r] -> Mux1/3
  Gain/1 -> a_b/1
  Data Type Conversion1/1 -> MATLAB Function/1(u)
  MATLAB Function/1(y) -> Gain/1
  MATLAB Function1/1(y) -> Gain1/1
  Gain1/1 -> w_b/1

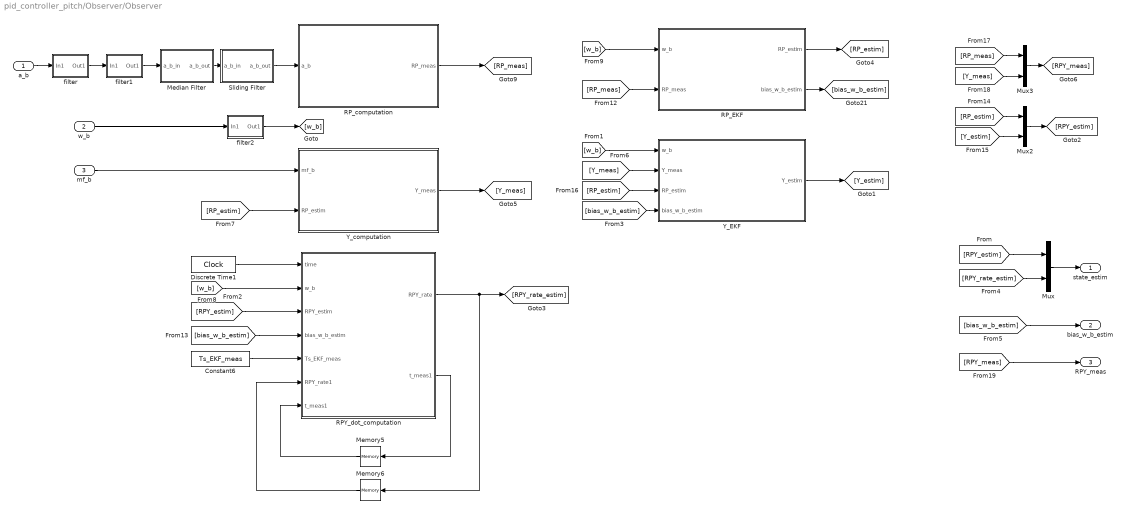
== system pid_controller_pitch/Observer/Observer ==
  a_b : Inport
  w_b : Inport  Port=2
  mf_b : Inport  Port=3
  " filter" : Subsystem  mask{p=5}
      mask prompts: p "pole (p)"
  " filter1" : Subsystem  mask{p=meas_pole}
      mask prompts: p "pole (p)"
  " filter2" : Subsystem  mask{p=meas_pole}
      mask prompts: p "pole (p)"
  Constant6 : Constant  Value=Ts_EKF_meas
  Discrete Time1 : DigitalClock  SampleTime=Ts_slk
  Median Filter : Subsystem
  Memory5 : Memory
  Memory6 : Memory
  Mux : Mux  Inputs=2
  Mux2 : Mux  Inputs=2
  Mux3 : Mux  Inputs=2
  RPY_dot_computation : MATLAB Function  TreatAsAtomicUnit=on
  RP_EKF : Subsystem
  RP_computation : MATLAB Function  TreatAsAtomicUnit=on
  Sliding Filter : Subsystem
  Y_EKF : Subsystem
  Y_computation : MATLAB Function  TreatAsAtomicUnit=on
  state_estim : Outport
  bias_w_b_estim : Outport  Port=2
  RPY_meas : Outport  Port=3
  wires:
  Memory5/1 -> RPY_dot_computation/7("t_meas1 ")
  Discrete Time1/1 -> RPY_dot_computation/1(time)
  RPY_dot_computation/2(t_meas1) -> Memory5/1
  [w_b] -> RPY_dot_computation/2(w_b)
  Memory6/1 -> RPY_dot_computation/6(RPY_rate1)
  RPY_dot_computation/1(RPY_rate) -> Memory6/1, [RPY_rate_estim]
  Constant6/1 -> RPY_dot_computation/5(Ts_EKF_meas)
  [RPY_estim] -> RPY_dot_computation/3(RPY_estim)
  [bias_w_b_estim] -> RPY_dot_computation/4(bias_w_b_estim)
  [RPY_estim] -> Mux/1
  [RPY_rate_estim] -> Mux/2
  Mux/1 -> state_estim/1
  [bias_w_b_estim] -> bias_w_b_estim/1
  [RPY_meas] -> RPY_meas/1
  RP_EKF/2(bias_w_b_estim) -> [bias_w_b_estim]
  [RP_estim] -> Y_computation/2(RP_estim)
  [Y_meas] -> Y_EKF/2(Y_meas)
  Y_computation/1(Y_meas) -> [Y_meas]
  RP_EKF/1(RP_estim) -> [RP_estim]
  [w_b] -> Y_EKF/1(w_b)
  RP_computation/1(RP_meas) -> [RP_meas]
  [RP_meas] -> RP_EKF/2(RP_meas)
  [w_b] -> RP_EKF/1(w_b)
  Y_EKF/1(Y_estim) -> [Y_estim]
  mf_b/1 -> Y_computation/1(mf_b)
  w_b/1 -> " filter2"/1(In1)
  [bias_w_b_estim] -> Y_EKF/4(bias_w_b_estim)
  [RP_estim] -> Mux2/1
  [Y_estim] -> Mux2/2
  Mux2/1 -> [RPY_estim]
  [RP_estim] -> Y_EKF/3(RP_estim)
  [RP_meas] -> Mux3/1
  Mux3/1 -> [RPY_meas]
  [Y_meas] -> Mux3/2
  Sliding Filter/1(a_b_out) -> RP_computation/1(a_b)
  Median Filter/1(a_b_out) -> Sliding Filter/1(a_b_in)
  " filter1"/1(Out1) -> Median Filter/1(a_b_in)
  " filter"/1(Out1) -> " filter1"/1(In1)
  a_b/1 -> " filter"/1(In1)
  " filter2"/1(Out1) -> [w_b]

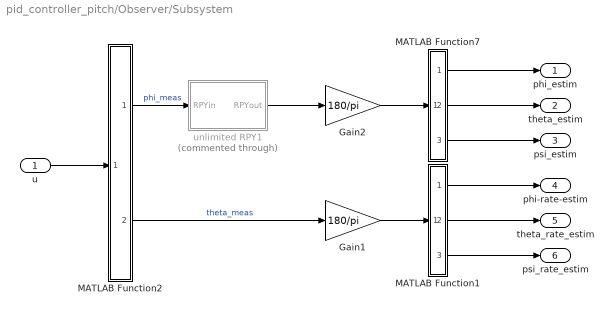
== system pid_controller_pitch/Observer/Subsystem ==
  u : Inport
  Gain1 : Gain  Gain=180/pi
  Gain2 : Gain  Gain=180/pi
  MATLAB Function1 : MATLAB Function  TreatAsAtomicUnit=on
  MATLAB Function2 : MATLAB Function  TreatAsAtomicUnit=on
  MATLAB Function7 : MATLAB Function  TreatAsAtomicUnit=on
  unlimited RPY1 : Subsystem  Commented=through
  phi_estim : Outport
  theta_estim : Outport  Port=2
  psi_estim : Outport  Port=3
  phi-rate-estim : Outport  Port=4
  theta_rate_estim : Outport  Port=5
  psi_rate_estim : Outport  Port=6
  wires:
  u/1 -> MATLAB Function2/1(u)
  MATLAB Function2/2(y2) -> Gain1/1  "theta_meas"
  MATLAB Function2/1(y1) -> unlimited RPY1/1(RPYin)  "phi_meas"
  MATLAB Function7/2(y2) -> theta_estim/1
  MATLAB Function7/1(y1) -> phi_estim/1
  MATLAB Function7/3(y3) -> psi_estim/1
  unlimited RPY1/1(RPYout) -> Gain2/1
  Gain2/1 -> MATLAB Function7/1(u)
  Gain1/1 -> MATLAB Function1/1(u)
  MATLAB Function1/3(y3) -> psi_rate_estim/1
  MATLAB Function1/2(y2) -> theta_rate_estim/1
  MATLAB Function1/1(y1) -> phi-rate-estim/1

== system pid_controller_pitch/Observer/unlimited RPY ==
  RPYin : Inport
  Memory : Memory
  Memory1 : Memory
  unlimited RPY : MATLAB Function  TreatAsAtomicUnit=on
  RPYout : Outport
  wires:
  RPYin/1 -> unlimited RPY/1("RPY ")
  unlimited RPY/1(RPY) -> Memory/1, RPYout/1
  Memory/1 -> unlimited RPY/2(RPY1)
  unlimited RPY/2(init) -> Memory1/1
  Memory1/1 -> unlimited RPY/3("init ")

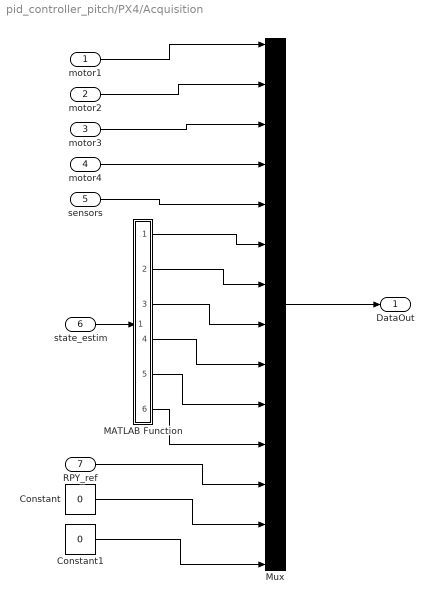
== system pid_controller_pitch/PX4/Acquisition ==
  motor1 : Inport
  motor2 : Inport  Port=2
  motor3 : Inport  Port=3
  motor4 : Inport  Port=4
  sensors : Inport  Port=5
  state_estim : Inport  Port=6
  RPY_ref : Inport  Port=7
  Constant : Constant  Value=0
  Constant1 : Constant  Value=0
  MATLAB Function : MATLAB Function  TreatAsAtomicUnit=on
  Mux : Mux  Inputs=14
  DataOut : Outport
  wires:
  state_estim/1 -> MATLAB Function/1(u)
  motor1/1 -> Mux/1
  motor2/1 -> Mux/2
  motor3/1 -> Mux/3
  motor4/1 -> Mux/4
  sensors/1 -> Mux/5
  MATLAB Function/1(y1) -> Mux/6
  MATLAB Function/2(y2) -> Mux/7
  MATLAB Function/3(y3) -> Mux/8
  MATLAB Function/4(y4) -> Mux/9
  MATLAB Function/5(y5) -> Mux/10
  MATLAB Function/6(y6) -> Mux/11
  Mux/1 -> DataOut/1
  RPY_ref/1 -> Mux/12
  Constant/1 -> Mux/13
  Constant1/1 -> Mux/14

== system pid_controller_pitch/PX4/U + BIAS ==
  u1 : Inport
  u2 : Inport  Port=2
  u3 : Inport  Port=3
  u4 : Inport  Port=4
  input1 : Subsystem
  input2 : Subsystem
  input3 : Subsystem
  input4 : Subsystem
  u1 + bias : Outport
  u2 + bias : Outport  Port=2
  u3 + bias : Outport  Port=3
  u4 + bias : Outport  Port=4
  wires:
  u2/1 -> input2/1(In1)
  u1/1 -> input1/1(In1)
  input1/1(Out1) -> u1 + bias/1
  u4/1 -> input4/1(In1)
  input4/1(Out1) -> u4 + bias/1
  input2/1(Out1) -> u2 + bias/1
  u3/1 -> input3/1(In1)
  input3/1(Out1) -> u3 + bias/1

== system pid_controller_pitch/Observer/Observer/ filter ==
  In1 : Inport
  Demux6 : Demux  Outputs=3
  Discrete Transfer Fcn : DiscreteTransferFcn  Numerator=[Ts_slk*p]  Denominator=[1 (Ts_slk*p-1)]
  Discrete Transfer Fcn1 : DiscreteTransferFcn  Numerator=[Ts_slk*p]  Denominator=[1 (Ts_slk*p-1)]
  Discrete Transfer Fcn2 : DiscreteTransferFcn  Numerator=[Ts_slk*p]  Denominator=[1 (Ts_slk*p-1)]
  Mux : Mux  Inputs=3
  Transfer Fcn1 : TransferFcn  Commented=on  Denominator=[1/p 1]
  Transfer Fcn3 : TransferFcn  Commented=on  Denominator=[1/p 1]
  Transfer Fcn4 : TransferFcn  Commented=on  Denominator=[1/p 1]
  Out1 : Outport
  wires:
  Discrete Transfer Fcn1/1 -> Mux/2
  Demux6/3 -> Discrete Transfer Fcn2/1
  Mux/1 -> Out1/1
  Discrete Transfer Fcn2/1 -> Mux/3
  Discrete Transfer Fcn/1 -> Mux/1
  In1/1 -> Demux6/1
  Demux6/1 -> Discrete Transfer Fcn/1
  Demux6/2 -> Discrete Transfer Fcn1/1

== system pid_controller_pitch/Observer/Observer/ filter1 ==
  In1 : Inport
  Demux6 : Demux  Outputs=3
  Discrete Transfer Fcn : DiscreteTransferFcn  Numerator=[Ts_slk*p]  Denominator=[1 (Ts_slk*p-1)]
  Discrete Transfer Fcn1 : DiscreteTransferFcn  Numerator=[Ts_slk*p]  Denominator=[1 (Ts_slk*p-1)]
  Discrete Transfer Fcn2 : DiscreteTransferFcn  Numerator=[Ts_slk*p]  Denominator=[1 (Ts_slk*p-1)]
  Mux : Mux  Inputs=3
  Transfer Fcn1 : TransferFcn  Commented=on  Denominator=[1/p 1]
  Transfer Fcn3 : TransferFcn  Commented=on  Denominator=[1/p 1]
  Transfer Fcn4 : TransferFcn  Commented=on  Denominator=[1/p 1]
  Out1 : Outport
  wires:
  Discrete Transfer Fcn1/1 -> Mux/2
  Demux6/3 -> Discrete Transfer Fcn2/1
  Mux/1 -> Out1/1
  Discrete Transfer Fcn2/1 -> Mux/3
  Discrete Transfer Fcn/1 -> Mux/1
  In1/1 -> Demux6/1
  Demux6/1 -> Discrete Transfer Fcn/1
  Demux6/2 -> Discrete Transfer Fcn1/1

== system pid_controller_pitch/Observer/Observer/ filter2 ==
  In1 : Inport
  Demux6 : Demux  Outputs=3
  Discrete Transfer Fcn : DiscreteTransferFcn  Numerator=[Ts_slk*p]  Denominator=[1 (Ts_slk*p-1)]
  Discrete Transfer Fcn1 : DiscreteTransferFcn  Numerator=[Ts_slk*p]  Denominator=[1 (Ts_slk*p-1)]
  Discrete Transfer Fcn2 : DiscreteTransferFcn  Numerator=[Ts_slk*p]  Denominator=[1 (Ts_slk*p-1)]
  Mux : Mux  Inputs=3
  Transfer Fcn1 : TransferFcn  Commented=on  Denominator=[1/p 1]
  Transfer Fcn3 : TransferFcn  Commented=on  Denominator=[1/p 1]
  Transfer Fcn4 : TransferFcn  Commented=on  Denominator=[1/p 1]
  Out1 : Outport
  wires:
  Discrete Transfer Fcn1/1 -> Mux/2
  Demux6/3 -> Discrete Transfer Fcn2/1
  Mux/1 -> Out1/1
  Discrete Transfer Fcn2/1 -> Mux/3
  Discrete Transfer Fcn/1 -> Mux/1
  In1/1 -> Demux6/1
  Demux6/1 -> Discrete Transfer Fcn/1
  Demux6/2 -> Discrete Transfer Fcn1/1

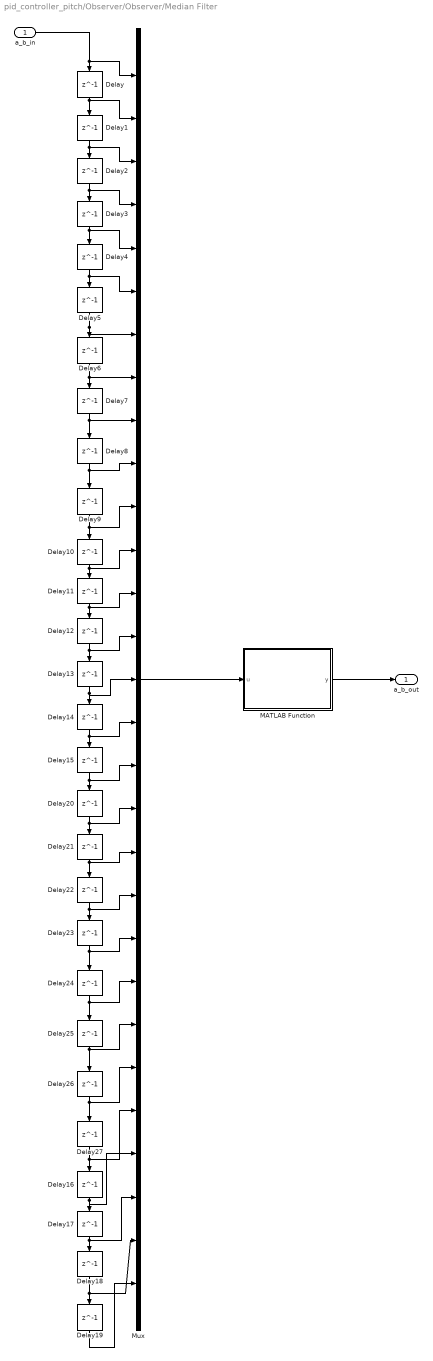
== system pid_controller_pitch/Observer/Observer/Median Filter ==
  a_b_in : Inport
  Delay{,1..27} (28 alike) : Delay  DelayLength=1  InitialCondition=zeros(1,3)  SampleTime=Ts_slk
  MATLAB Function : MATLAB Function  TreatAsAtomicUnit=on
  Mux : Mux  Inputs=29
  a_b_out : Outport
  wires:
  a_b_in/1 -> Delay/1, Mux/1
  Delay1/1 -> Delay2/1, Mux/3
  Delay2/1 -> Delay3/1, Mux/4
  Delay/1 -> Delay1/1, Mux/2
  Delay3/1 -> Delay4/1, Mux/5
  Mux/1 -> MATLAB Function/1(u)
  MATLAB Function/1(y) -> a_b_out/1
  Delay4/1 -> Delay5/1, Mux/6
  Delay5/1 -> Delay6/1, Mux/7
  Delay6/1 -> Delay7/1, Mux/8
  Delay8/1 -> Mux/10, Delay9/1
  Delay11/1 -> Mux/13, Delay12/1
  Delay12/1 -> Mux/14, Delay13/1
  Delay7/1 -> Mux/9, Delay8/1
  Delay9/1 -> Delay10/1, Mux/11
  Delay10/1 -> Mux/12, Delay11/1
  Delay13/1 -> Mux/15, Delay14/1
  Delay24/1 -> Mux/22, Delay25/1
  Delay23/1 -> Mux/21, Delay24/1
  Delay20/1 -> Mux/18, Delay21/1
  Delay15/1 -> Mux/17, Delay20/1
  Delay21/1 -> Mux/19, Delay22/1
  Delay27/1 -> Mux/25, Delay16/1
  Delay18/1 -> Delay19/1, Mux/28
  Delay25/1 -> Mux/23, Delay26/1
  Delay22/1 -> Mux/20, Delay23/1
  Delay26/1 -> Mux/24, Delay27/1
  Delay14/1 -> Mux/16, Delay15/1
  Delay17/1 -> Mux/27, Delay18/1
  Delay16/1 -> Mux/26, Delay17/1
  Delay19/1 -> Mux/29

== system pid_controller_pitch/Observer/Observer/RP_EKF ==
  w_b : Inport
  RP_meas : Inport  Port=2
  Delay2 : Delay  DelayLength=1  SampleTime=Ts_EKF_meas
  Discrete Time : DigitalClock  SampleTime=Ts_slk
  EKF_RP : MATLAB Function  TreatAsAtomicUnit=on
  MATLAB Function : MATLAB Function  TreatAsAtomicUnit=on
  Memory2 : Memory
  Memory3 : Memory  InitialCondition=P0_phth
  Memory4 : Memory  InitialCondition=x0_phth
  RP_estim : Outport
  bias_w_b_estim : Outport  Port=2
  wires:
  w_b/1 -> Delay2/1
  EKF_RP/2(Pk) -> Memory3/1
  Memory2/1 -> EKF_RP/6("t_meas ")
  EKF_RP/3(t_meas) -> Memory2/1
  RP_meas/1 -> EKF_RP/5(RP_meas)
  Discrete Time/1 -> EKF_RP/1(time)
  Memory3/1 -> EKF_RP/3(Pk1)
  Delay2/1 -> EKF_RP/4(w_b1)
  Memory4/1 -> EKF_RP/2(xk1)
  EKF_RP/1(xk) -> Memory4/1, MATLAB Function/1(xk)  "xk"
  MATLAB Function/1(RP_estim) -> RP_estim/1
  MATLAB Function/2(bias_w_b_estim) -> bias_w_b_estim/1

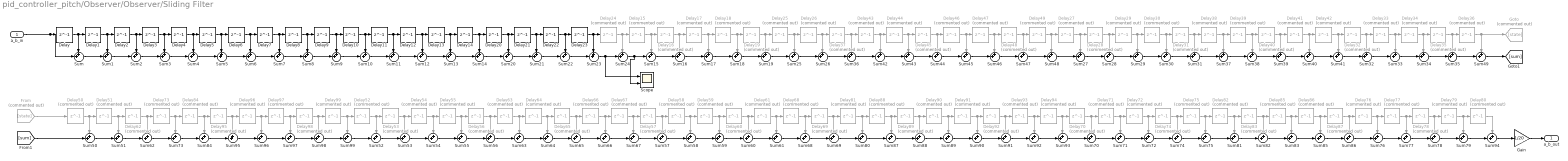
== system pid_controller_pitch/Observer/Observer/Sliding Filter ==
  a_b_in : Inport
  Delay{,1..14,20..23} (19 alike) : Delay  DelayLength=1  SampleTime=Ts_slk
  Delay{15..19,24..99} (81 alike) : Delay  Commented=on  DelayLength=1  SampleTime=Ts_slk
  From : From  Commented=on  GotoTag=state
  Gain : Gain  Gain=1/20
  Goto : Goto  Commented=on  GotoTag=state
  Scope : Scope  NumInputPorts=2
  Sum{,1..99} (100 alike) : Sum  Inputs=++|
  a_b_out : Outport
  wires:
  Delay/1 -> Sum/1, Delay1/1
  Delay1/1 -> Sum1/1, Delay2/1
  Delay2/1 -> Sum2/1, Delay3/1
  Delay3/1 -> Sum3/1, Delay4/1
  Sum/1 -> Sum1/2
  Sum1/1 -> Sum2/2
  Sum2/1 -> Sum3/2
  Sum3/1 -> Sum4/2
  Delay4/1 -> Delay5/1, Sum4/1
  Sum4/1 -> Sum5/2
  a_b_in/1 -> Sum/2, Delay/1
  Delay5/1 -> Sum5/1, Delay6/1
  Delay6/1 -> Sum6/1, Delay7/1
  Sum5/1 -> Sum6/2
  Sum6/1 -> Sum7/2
  Sum7/1 -> Sum8/2
  Delay7/1 -> Sum7/1, Delay8/1
  Delay8/1 -> Delay9/1, Sum8/1
  Delay9/1 -> Sum9/1, Delay10/1
  Delay10/1 -> Sum10/1, Delay11/1
  Delay11/1 -> Sum11/1, Delay12/1
  Delay12/1 -> Sum12/1, Delay13/1
  Delay13/1 -> Sum13/1, Delay14/1
  Sum11/1 -> Sum12/2
  Sum12/1 -> Sum13/2
  Sum13/1 -> Sum14/2
  Sum8/1 -> Sum9/2
  Sum9/1 -> Sum10/2
  Sum10/1 -> Sum11/2
  Delay14/1 -> Delay20/1, Sum14/1
  Delay19/1 -> Delay25/1, Sum19/1
  Sum16/1 -> Sum17/2
  Delay15/1 -> Sum15/1, Delay16/1
  Sum24/1 -> Scope/2, Sum15/2
  Sum17/1 -> Sum18/2
  Delay23/1 -> Delay24/1, Sum23/1
  Delay24/1 -> Sum24/1, Delay15/1
  Sum20/1 -> Sum21/2
  Delay22/1 -> Sum22/1, Delay23/1
  Delay18/1 -> Sum18/1, Delay19/1
  Sum23/1 -> Scope/1, Sum24/2
  Sum22/1 -> Sum23/2
  Sum14/1 -> Sum20/2
  Delay20/1 -> Sum20/1, Delay21/1
  Delay17/1 -> Sum17/1, Delay18/1
  Sum18/1 -> Sum19/2
  Delay21/1 -> Sum21/1, Delay22/1
  Delay16/1 -> Sum16/1, Delay17/1
  Sum15/1 -> Sum16/2
  Sum21/1 -> Sum22/2
  Sum41/1 -> Sum32/2
  Delay32/1 -> Sum32/1, Delay33/1
  Sum33/1 -> Sum34/2
  Delay42/1 -> Sum41/1, Delay32/1
  Sum37/1 -> Sum38/2
  Delay41/1 -> Delay42/1, Sum40/1
  Delay31/1 -> Delay38/1, Sum31/1
  Sum28/1 -> Sum29/2
  Delay28/1 -> Sum28/1, Delay29/1
  Delay27/1 -> Sum27/1, Delay28/1
  Delay49/1 -> Sum48/1, Delay27/1
  Sum48/1 -> Sum27/2
  Sum29/1 -> Sum30/2
  Delay48/1 -> Delay49/1, Sum47/1
  Sum44/1 -> Sum45/2
  Delay47/1 -> Sum46/1, Delay48/1
  Delay45/1 -> Sum44/1, Delay46/1
  Delay39/1 -> Sum38/1, Delay40/1
  Sum47/1 -> Sum48/2
  Delay38/1 -> Sum37/1, Delay39/1
  Sum40/1 -> Sum41/2
  Sum46/1 -> Sum47/2
  Sum34/1 -> Sum35/2
  Delay29/1 -> Sum29/1, Delay30/1
  Sum32/1 -> Sum33/2
  Delay40/1 -> Sum39/1, Delay41/1
  Delay46/1 -> Sum45/1, Delay47/1
  Delay33/1 -> Sum33/1, Delay34/1
  Sum27/1 -> Sum28/2
  Delay30/1 -> Sum30/1, Delay31/1
  Sum36/1 -> Sum42/2
  Delay44/1 -> Delay45/1, Sum43/1
  Sum39/1 -> Sum40/2
  Delay37/1 -> Sum36/1, Delay43/1
  Sum26/1 -> Sum36/2
  Sum43/1 -> Sum44/2
  Sum25/1 -> Sum26/2
  Delay35/1 -> Sum35/1, Delay36/1
  Sum42/1 -> Sum43/2
  Delay43/1 -> Sum42/1, Delay44/1
  Sum30/1 -> Sum31/2
  Sum45/1 -> Sum46/2
  Sum31/1 -> Sum37/2
  Delay26/1 -> Sum26/1, Delay37/1
  Delay25/1 -> Sum25/1, Delay26/1
  Delay34/1 -> Sum34/1, Delay35/1
  Sum38/1 -> Sum39/2
  Sum35/1 -> Sum49/2
  Sum19/1 -> Sum25/2
  Delay36/1 -> Goto/1, Sum49/1
  Sum49/1 -> [sum]
  Delay68/1 -> Sum68/1, Delay69/1
  Sum82/1 -> Sum83/2
  Sum68/1 -> Sum69/2
  Sum75/1 -> Sum81/2
  Delay88/1 -> Sum87/1, Delay89/1
  Delay79/1 -> Sum79/1, Delay80/1
  Sum74/1 -> Sum75/2
  Delay69/1 -> Sum69/1, Delay81/1
  Sum90/1 -> Sum91/2
  Sum83/1 -> Sum85/2
  Sum80/1 -> Sum87/2
  Sum88/1 -> Sum89/2
  Sum69/1 -> Sum80/2
  Sum70/1 -> Sum71/2
  Delay78/1 -> Sum78/1, Delay79/1
  Sum92/1 -> Sum93/2
  Sum78/1 -> Sum79/2
  Sum91/1 -> Sum92/2
  Sum85/1 -> Sum86/2
  Sum76/1 -> Sum77/2
  Delay72/1 -> Sum72/1, Delay74/1
  Delay82/1 -> Sum81/1, Delay83/1
  Sum72/1 -> Sum74/2
  Delay94/1 -> Sum93/1, Delay70/1
  Delay85/1 -> Sum83/1, Delay86/1
  Delay74/1 -> Sum74/1, Delay75/1
  Sum93/1 -> Sum70/2
  Delay90/1 -> Sum89/1, Delay91/1
  Delay92/1 -> Sum91/1, Delay93/1
  Delay93/1 -> Delay94/1, Sum92/1
  Delay75/1 -> Delay82/1, Sum75/1
  Sum71/1 -> Sum72/2
  Delay71/1 -> Sum71/1, Delay72/1
  Delay70/1 -> Sum70/1, Delay71/1
  Sum67/1 -> Sum57/2
  Delay57/1 -> Sum57/1, Delay58/1
  Sum58/1 -> Sum59/2
  Sum89/1 -> Sum90/2
  Delay61/1 -> Delay68/1, Sum61/1
  Delay67/1 -> Sum67/1, Delay57/1
  Sum63/1 -> Sum64/2
  Delay66/1 -> Delay67/1, Sum66/1
  Sum94/1 -> Gain/1
  Sum81/1 -> Sum82/2
  Sum77/1 -> Sum78/2
  Delay87/1 -> Sum86/1, Delay76/1
  Delay76/1 -> Sum76/1, Delay77/1
  Delay86/1 -> Delay87/1, Sum85/1
  Sum86/1 -> Sum76/2
  Sum53/1 -> Sum54/2
  Delay53/1 -> Sum53/1, Delay54/1
  Delay56/1 -> Delay63/1, Sum56/1
  Delay52/1 -> Sum52/1, Delay53/1
  Delay99/1 -> Sum99/1, Delay52/1
  Sum99/1 -> Sum52/2
  Sum54/1 -> Sum55/2
  Delay98/1 -> Delay99/1, Sum98/1
  Sum95/1 -> Sum96/2
  Delay97/1 -> Sum97/1, Delay98/1
  Delay95/1 -> Sum95/1, Delay96/1
  Delay55/1 -> Sum55/1, Delay56/1
  Sum98/1 -> Sum99/2
  Sum64/1 -> Sum65/2
  Delay64/1 -> Sum64/1, Delay65/1
  Delay58/1 -> Sum58/1, Delay59/1
  Delay81/1 -> Sum80/1, Delay88/1
  Delay63/1 -> Sum63/1, Delay64/1
  Sum66/1 -> Sum67/2
  Sum97/1 -> Sum98/2
  Delay77/1 -> Sum77/1, Delay78/1
  Sum59/1 -> Sum60/2
  Delay54/1 -> Sum54/1, Delay55/1
  Sum57/1 -> Sum58/2
  Delay89/1 -> Delay90/1, Sum88/1
  Delay65/1 -> Sum65/1, Delay66/1
  Delay96/1 -> Sum96/1, Delay97/1
  Sum52/1 -> Sum53/2
  From/1 -> Delay50/1
  Delay83/1 -> Sum82/1, Delay85/1
  Sum62/1 -> Sum73/2
  Delay84/1 -> Delay95/1, Sum84/1
  Sum65/1 -> Sum66/2
  Sum87/1 -> Sum88/2
  Delay62/1 -> Sum62/1, Delay73/1
  Sum51/1 -> Sum62/2
  Delay91/1 -> Sum90/1, Delay92/1
  Sum84/1 -> Sum95/2
  Sum50/1 -> Sum51/2
  Delay60/1 -> Sum60/1, Delay61/1
  Sum73/1 -> Sum84/2
  Delay73/1 -> Sum73/1, Delay84/1
  Sum55/1 -> Sum56/2
  Sum61/1 -> Sum68/2
  Delay80/1 -> Sum94/1
  Sum96/1 -> Sum97/2
  Sum79/1 -> Sum94/2
  Sum56/1 -> Sum63/2
  Delay51/1 -> Sum51/1, Delay62/1
  Delay50/1 -> Sum50/1, Delay51/1
  Delay59/1 -> Sum59/1, Delay60/1
  Sum60/1 -> Sum61/2
  Gain/1 -> a_b_out/1
  [sum] -> Sum50/2

== system pid_controller_pitch/Observer/Observer/Y_EKF ==
  w_b : Inport
  Y_meas : Inport  Port=2
  RP_estim : Inport  Port=3
  bias_w_b_estim : Inport  Port=4
  Delay2 : Delay  DelayLength=1  SampleTime=Ts_EKF_meas
  Discrete Time : DigitalClock  SampleTime=Ts_slk
  EKF_Y : MATLAB Function  TreatAsAtomicUnit=on
  Memory2 : Memory
  Memory3 : Memory  InitialCondition=ones(1,1)*P0_ps
  Memory4 : Memory  InitialCondition=ones(1,1)*x0_ps
  Y_estim : Outport
  wires:
  w_b/1 -> Delay2/1
  EKF_Y/2(Pk) -> Memory3/1  "Pk"
  Memory2/1 -> EKF_Y/8("t_meas ")
  EKF_Y/3(t_meas) -> Memory2/1  "t_meas"
  Y_meas/1 -> EKF_Y/5(Y_meas)
  Discrete Time/1 -> EKF_Y/1(time)
  Memory3/1 -> EKF_Y/3(Pk1)
  Delay2/1 -> EKF_Y/4(w_b1)
  Memory4/1 -> EKF_Y/2(xk1)
  EKF_Y/1(xk) -> Memory4/1, Y_estim/1  "xk"
  bias_w_b_estim/1 -> EKF_Y/7(bias_w_b_estim)
  RP_estim/1 -> EKF_Y/6(RP_estim)

== system pid_controller_pitch/Observer/Subsystem/unlimited RPY1 ==
  RPYin : Inport
  Memory : Memory
  Memory1 : Memory
  unlimited RPY : MATLAB Function  TreatAsAtomicUnit=on
  RPYout : Outport
  wires:
  RPYin/1 -> unlimited RPY/1("RPY ")
  unlimited RPY/1(RPY) -> Memory/1, RPYout/1
  Memory/1 -> unlimited RPY/2(RPY1)
  unlimited RPY/2(init) -> Memory1/1
  Memory1/1 -> unlimited RPY/3("init ")

== system pid_controller_pitch/PX4/U + BIAS/input1 ==
  In1 : Inport
  Constant : Constant  Value=1000  SampleTime=0.01
  Data Type Conversion1 : DataTypeConversion  OutDataTypeStr=uint16  SaturateOnIntegerOverflow=off  RndMeth=Floor
  Sum : Sum  Inputs=|++
  Out1 : Outport
  wires:
  Sum/1 -> Data Type Conversion1/1
  In1/1 -> Sum/1
  Constant/1 -> Sum/2
  Data Type Conversion1/1 -> Out1/1

== system pid_controller_pitch/PX4/U + BIAS/input2 ==
  In1 : Inport
  Constant : Constant  Value=1000  SampleTime=0.01
  Data Type Conversion1 : DataTypeConversion  OutDataTypeStr=uint16  SaturateOnIntegerOverflow=off  RndMeth=Floor
  Sum : Sum  Inputs=|++
  Out1 : Outport
  wires:
  Sum/1 -> Data Type Conversion1/1
  In1/1 -> Sum/1
  Constant/1 -> Sum/2
  Data Type Conversion1/1 -> Out1/1

== system pid_controller_pitch/PX4/U + BIAS/input3 ==
  In1 : Inport
  Constant : Constant  Value=1000  SampleTime=0.01
  Data Type Conversion1 : DataTypeConversion  OutDataTypeStr=uint16  SaturateOnIntegerOverflow=off  RndMeth=Floor
  Sum : Sum  Inputs=|++
  Out1 : Outport
  wires:
  Sum/1 -> Data Type Conversion1/1
  In1/1 -> Sum/1
  Constant/1 -> Sum/2
  Data Type Conversion1/1 -> Out1/1

== system pid_controller_pitch/PX4/U + BIAS/input4 ==
  In1 : Inport
  Constant : Constant  Value=1000  SampleTime=0.01
  Data Type Conversion1 : DataTypeConversion  OutDataTypeStr=uint16  SaturateOnIntegerOverflow=off  RndMeth=Floor
  Sum : Sum  Inputs=|++
  Out1 : Outport
  wires:
  Sum/1 -> Data Type Conversion1/1
  In1/1 -> Sum/1
  Constant/1 -> Sum/2
  Data Type Conversion1/1 -> Out1/1

== matlab function pid_controller_pitch/MATLAB Function3 ==
  data: u input; y1 output; y2 output; y3 output
function [y1,y2,y3] = fcn(u)

y1 = u(1);
y2 = u(2);
y3 = u(3);

== matlab function pid_controller_pitch/Observer/Observer/RP_EKF/MATLAB Function ==
  data: xk input; RP_estim output; bias_w_b_estim output
function [RP_estim, bias_w_b_estim] = state_extraction(xk)

RP_estim        = xk(1:2,1);
bias_w_b_estim  = xk(3:5,1);
end

== matlab function pid_controller_pitch/Observer/MATLAB Function1 ==
  data: u input; y1 output; y2 output; y3 output
function [y1,y2,y3] = fcn(u)

y1 = u(1);
y2 = u(2);
y3 = u(3);

== matlab function pid_controller_pitch/Observer/IMU measurements & rotation/MATLAB Function ==
  data: u input; y output
function y = a_b_roation(u)
y = zeros(3,1);
y(1) = -u(1);
y(2) = +u(2);
y(3) = +u(3);
end

== matlab function pid_controller_pitch/Observer/Observer/RPY_dot_computation ==
  data: time input; w_b input; RPY_estim input; bias_w_b_estim input; Ts_EKF_meas input; RPY_rate1 input; RPY_rate output; t_meas1 input; t_meas1 output
function [RPY_rate,t_meas1] = RPY_dot_computation(time,w_b,RPY_estim,bias_w_b_estim,Ts_EKF_meas,RPY_rate1,t_meas1)

if time - t_meas1 >= Ts_EKF_meas || time == 0
    wp          =       w_b(1,1);               % p-dir of angular velocity w
    wq          =       w_b(2,1);               % q-dir of angular velocity w
    wr          =       w_b(3,1);               % r-dir of angular velocity w

    phi         =       RPY_estim(1,1);         % roll angle (rad)
    theta       =       RPY_estim(2,1);         % pitch angle (rad)
    psi         =       RPY_estim(3,1);         % yaw angle (rad)  
    bias_wp     =       bias_w_b_estim(1,1)*0;    % bias of p-dir of angular velocity w
    bias_wq     =       bias_w_b_estim(2,1)*0;    % bias of q-dir of angular velocity w
    bias_wr     =       bias_w_b_estim(3,1)*0;   % bias of r-dir of angular velocity w

    cph         =       cos(phi);
    cth         =       cos(theta);
    cps         =       cos(psi);
    sph         =       sin(phi);
    sth         =       sin(theta);
    sps         =       sin(psi);
    tth         =       sth/cth;

    % integration step
    t_meas1 = time;
    W_eta = [1,    sph*tth,    cph*tth;
             0,    cph,        -sph;
             0,    sph/cth,    cph/cth;];
    w_b_corrected = [wp-bias_wp; wq-bias_wq; wr-bias_wr;];
    RPY_rate = W_eta*w_b_corrected;
else
    RPY_rate = RPY_rate1;
end
end

== matlab function pid_controller_pitch/Sensors/correct sequence ==
  data: u input; y output
function y  = fcn(u)

y = single([0,0,0]);
y(1) = u(3);
y(2) = u(2);
y(3) = u(1);

== matlab function pid_controller_pitch/Observer/Subsystem/MATLAB Function2 ==
  data: u input; y1 output; y2 output
function [y1,y2] = fcn(u)

y1 = u(1:3);
y2 = u(4:6);
end

== matlab function pid_controller_pitch/Controller Camilla/MATLAB Function1 ==
  data: x1 input; x output; u_sat1 input; e input; u_sat output; A_cond parameter; B_cond parameter; C parameter; D parameter; u_min input; u_max input; on_off input
function [x,u_sat]= PID_controller(x1,u_sat1,e, A_cond, B_cond, C, D, u_min, u_max, on_off)
if on_off == 0
    x1 = zeros(2,1);
    u_sat1 = 0;
end
x       =   A_cond*x1 + B_cond*u_sat1;
u       =   C*x + D*e;
u_sat   =   max(u_min, min (u_max, u));  
end

== matlab function pid_controller_pitch/Controller 1dof/MATLAB Function3 ==
  data: tau input; tau_o output
function tau_o=fcn(tau)
% Inputs:   tau    (torque 1x1)         
%
% Outputs:  tau_o  (torque 3x1)

% States in input
tau_1     =       tau(1,1);     %  roll torque

% States in output
tau_o      =       zeros(3,1);
tau_o(1,1) =       tau_1;   
tau_o(2,1) =       0;
tau_o(3,1) =       0;

== matlab function pid_controller_pitch/MATLAB Function2 ==
  data: u_vect input; u1 output; u2 output; u3 output; u4 output
function [u1,u2,u3,u4] = fcn(u_vect)

u1 = u_vect(1);
u2 = u_vect(2);
u3 = u_vect(3);
u4 = u_vect(4);
end

== matlab function pid_controller_pitch/allocation_logic ==
  data: tau input; u_max input; u output; tau_allocated output; u_min input; param parameter
function [u, tau_allocated] = allocation_logic(tau,u_max,u_min,param)
% Allocation Logic Block: computes the corresponding control command
% u = [u1,u2,u3,u4] given the torque command tau = [tau_phi, tau_theta, tau_phi]

% control command limits
%%u_min = 100;
% u_max = 1000;

l  = param(4,1);
k1 = param(5,1);
k2 = param(6,1);
k3 = param(7,1);
k4 = param(8,1);
b  = param(9,1);

u = zeros(4,1);
% [tau_ph; tau_th; tau_ps] = Mtau_u * [u1;u2;u3;u4]
Mtau_u = [0       0        l*k3    -l*k4;
         -l*k1    l*k2     0        0;
         -b      -b        b        b;];
% Minv = Mtau_u'*inv(Mtau_u*Mtau_u');
% up = Minv*tau;
% un = zeros(4,1);
% if min(up(:)) < u_min 
%     un = ones(4,1)*(u_min - min(up(:)));
% end
% u = up+un;
% for i = 1:1:4
%     if u(i,1) > u_max
%         u(i,1) = u_max;
%     end
% end
if tau(1) >= 0
    u(4) = u_min;
    u(3) = (tau(1) + l*k4*u(4))/(l*k3);
else
    u(3) = u_min;
    u(4) = (-tau(1) + l*k3*u(3))/(l*k4);
end
if tau(2) >= 0
    u(1) = u_min;
    u(2) = (tau(2) + l*k1*u(1))/(l*k2);
else
    u(2) = u_min;
    u(1) = (-tau(2) + l*k2*u(2))/(l*k1);
end
u = min(u_max,u);
tau_allocated = Mtau_u*u;

== matlab function pid_controller_pitch/Observer/Observer/Median Filter/MATLAB Function ==
  data: u input; y output
function y = fcn(u)
[n,~] = size(u);
n = n/3;
norm = zeros(n,2);
for i = 1:1:n
    u_vect      = u(i*3-2:i*3,1); 
    norm(i,1)   = sqrt(u_vect'*u_vect);     % norm
    norm(i,2)   = i;                        % index
end
for i = 1:n-1
    for j = 1:n-i
        if norm(j,1) > norm(j+1,1)
            % Swap elements
            temp = norm(j,:);
            norm(j,:) = norm(j+1,:);
            norm(j+1,:) = temp;
        end
    end
end
indexMedian = floor(n/2-1);
median = norm(indexMedian,2);
y = u(median*3-2:median*3);
end

== matlab function pid_controller_pitch/Controller Camilla/MATLAB Function3 ==
  data: tau input; tau_o output
function tau_o=fcn(tau)
% Inputs:   tau    (torque 1x1)         
%
% Outputs:  tau_o  (torque 3x1)

% States in input
tau_2     =       tau(1,1);     %  roll torque

% States in output
tau_o      =       zeros(3,1);
tau_o(1,1) =       0;   
tau_o(2,1) =       tau_2;
tau_o(3,1) =       0;
